simulink model "Two_r"  (R2020a)
settings: Solver=VariableStepAuto  StartTime=0.0  StopTime=stoptime  RelTol=1e-3
undefined symbols (not defined in the file or in its folder): A, b, ct, M_inv, M_N, x0
settings Model: Creator=SURAJ  LastModifiedBy=shita
settings DataIOCC: ReturnWorkspaceOutputs=off
settings DebuggingCC: ArithmeticOperatorsInVariantConditions=warning
settings SFSimCC: SimUseLocalCustomCode=off  CustomCodeUndefinedFunction=UseInterfaceOnly
settings RTWCC: RTWUseLocalCustomCode=off

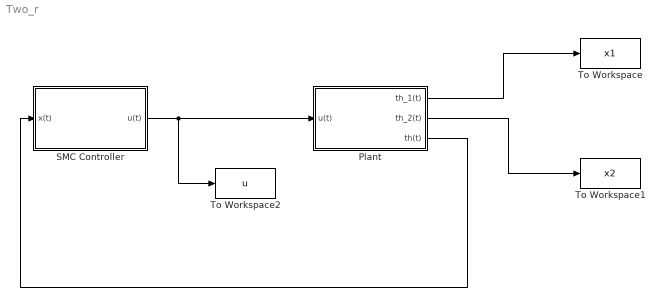
== system Two_r ==
  Plant : Subsystem
  SMC Controller : Subsystem
  To Workspace : ToWorkspace  VariableName=x1  SaveFormat=Timeseries  SampleTime=-1
  To Workspace1 : ToWorkspace  VariableName=x2  SaveFormat=Timeseries  SampleTime=-1
  To Workspace2 : ToWorkspace  VariableName=u  SaveFormat=Timeseries  SampleTime=-1
  wires:
  Plant/3(th(t)) -> SMC Controller/1(x(t))
  Plant/1(th_1(t)) -> To Workspace/1
  Plant/2(th_2(t)) -> To Workspace1/1
  SMC Controller/1(u(t)) -> To Workspace2/1, Plant/1(u(t))

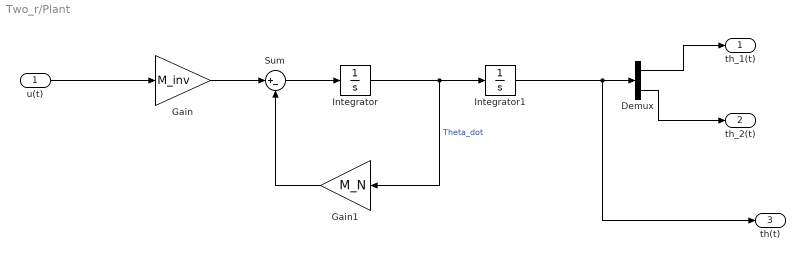
== system Two_r/Plant ==
  u(t) : Inport
  Demux : Demux  Outputs=2
  Gain : Gain  Gain=M_inv
  Gain1 : Gain  Gain=M_N
  Integrator : Integrator  InitialCondition=x0
  Integrator1 : Integrator  InitialCondition=x0
  Sum : Sum  Inputs=|+-
  th_1(t) : Outport  VectorParamsAs1DForOutWhenUnconnected=off
  th_2(t) : Outport  Port=2  VectorParamsAs1DForOutWhenUnconnected=off
  th(t) : Outport  Port=3  VectorParamsAs1DForOutWhenUnconnected=off
  wires:
  Demux/1 -> th_1(t)/1
  Demux/2 -> th_2(t)/1
  Integrator/1 -> Gain1/1, Integrator1/1  "Theta_dot"
  Integrator1/1 -> th(t)/1, Demux/1
  Gain/1 -> Sum/1
  Gain1/1 -> Sum/2
  Sum/1 -> Integrator/1
  u(t)/1 -> Gain/1

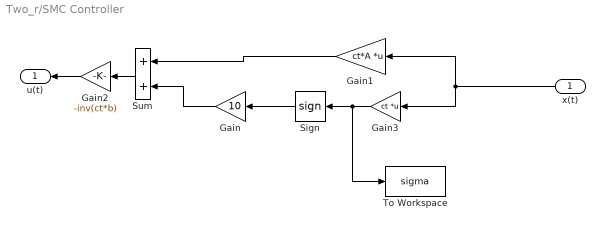
== system Two_r/SMC Controller ==
  x(t) : Inport
  Gain : Gain  Gain=10
  Gain1 : Gain  Gain=ct*A  Multiplication=Matrix(K*u) (u vector)
  Gain2 : Gain  Gain=-inv(ct*b)
  Gain3 : Gain  Gain=ct  Multiplication=Matrix(K*u) (u vector)
  Sign : Signum  ZeroCross=off
  Sum : Sum
  To Workspace : ToWorkspace  VariableName=sigma  SaveFormat=Timeseries  SampleTime=-1
  u(t) : Outport  VectorParamsAs1DForOutWhenUnconnected=off
  wires:
  Gain2/1 -> u(t)/1
  Gain/1 -> Sum/2
  Sum/1 -> Gain2/1
  Sign/1 -> Gain/1
  Gain1/1 -> Sum/1
  Gain3/1 -> Sign/1, To Workspace/1
  x(t)/1 -> Gain1/1, Gain3/1
